simulink model "fig9"  (R2023b)
settings: Solver=VariableStepAuto  StartTime=0.0  StopTime=10.0  RelTol=1e-3
libraries: fuzblock x2
settings Model: Creator=yusuf  LastModifiedBy=yusuf

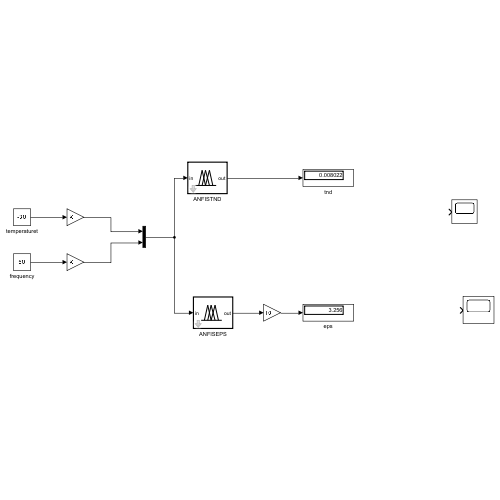
[thumbnail: Simulink's stored preview of the top-level diagram]
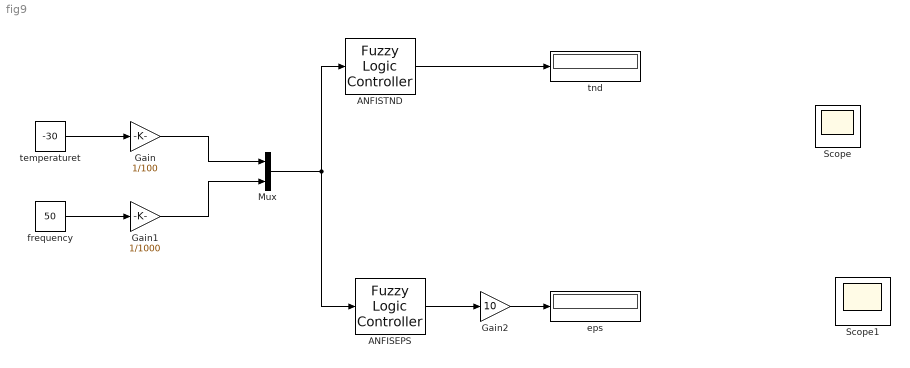
== system fig9 ==
  ANFISEPS : fuzblock/Fuzzy Logic  Controller  FIS=md55  OutputSampleNumber=101  DataType=double  FuzzifiedInputs=off  RuleFiringStrengths=off  RuleOutputs=off  AggregatedOutputs=off  SimulateUsing=Interpreted execution  OutOfRangeInputValueMessage=warning  NoRuleFiredMessage=warning  EmptyOutputFuzzySetMessage=warning
  ANFISTND : fuzblock/Fuzzy Logic  Controller  FIS=md155  OutputSampleNumber=101  DataType=double  FuzzifiedInputs=off  RuleFiringStrengths=off  RuleOutputs=off  AggregatedOutputs=off  SimulateUsing=Interpreted execution  OutOfRangeInputValueMessage=warning  NoRuleFiredMessage=warning  EmptyOutputFuzzySetMessage=warning
  Gain : Gain  Gain=1/100
  Gain1 : Gain  Gain=1/1000
  Gain2 : Gain  Gain=10
  Mux : Mux  Inputs=2
  Scope : Scope
  Scope1 : Scope
  eps : Display
  frequency : Constant  Value=50
  temperaturet : Constant  Value=-30
  tnd : Display
  wires:
  Mux/1 -> ANFISEPS/1, ANFISTND/1
  temperaturet/1 -> Gain/1
  frequency/1 -> Gain1/1
  ANFISTND/1 -> tnd/1
  Gain/1 -> Mux/1
  Gain1/1 -> Mux/2
  ANFISEPS/1 -> Gain2/1
  Gain2/1 -> eps/1
